simulink library "hysteresis_rods"  (R2016b)
settings: Solver=VariableStepAuto  StartTime=0.0  StopTime=10.0  RelTol=1e-3
undefined symbols (not defined in the file or in its folder): sim_params
libraries: hysteresis_curve x2, aerolibutil x1
settings Model: Creator=Sean  LastModifiedBy=bijan

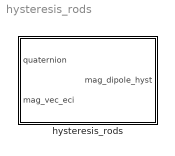
== system hysteresis_rods ==
  hysteresis_rods : Subsystem

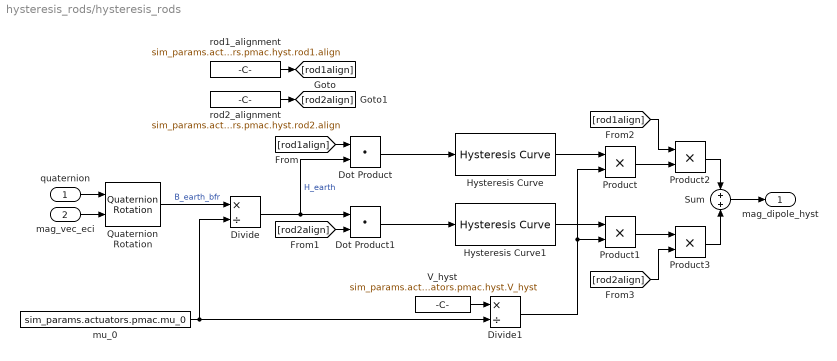
== system hysteresis_rods/hysteresis_rods ==
  quaternion : Inport
  mag_vec_eci : Inport  Port=2
  Divide : Product  Inputs=*/
  Divide1 : Product  Inputs=*/
  Dot Product : DotProduct  InputSameDT=on  OutDataTypeStr=Inherit: Inherit via internal rule
  Dot Product1 : DotProduct  InputSameDT=on  OutDataTypeStr=Inherit: Inherit via internal rule
  Hysteresis Curve : hysteresis_curve/Hysteresis Curve
  Hysteresis Curve1 : hysteresis_curve/Hysteresis Curve
  Product{,1..3} (4 alike) : Product
  Quaternion Rotation : aerolibutil/Quaternion Rotation
  Sum : Sum
  V_hyst : Constant  Value=sim_params.actuators.pmac.hyst.V_hyst
  mu_0 : Constant  Value=sim_params.actuators.pmac.mu_0
  rod1_alignment : Constant  Value=sim_params.actuators.pmac.hyst.rod1.align
  rod2_alignment : Constant  Value=sim_params.actuators.pmac.hyst.rod2.align
  mag_dipole_hyst : Outport
  wires:
  quaternion/1 -> Quaternion Rotation/1
  mag_vec_eci/1 -> Quaternion Rotation/2
  mu_0/1 -> Divide1/2, Divide/2
  Quaternion Rotation/1 -> Divide/1  "B_earth_bfr"
  V_hyst/1 -> Divide1/1
  Hysteresis Curve/1 -> Product/1
  Divide1/1 -> Product1/2, Product/2
  Divide/1 -> Dot Product1/1, Dot Product/2  "H_earth"
  Dot Product/1 -> Hysteresis Curve/1
  Dot Product1/1 -> Hysteresis Curve1/1
  Hysteresis Curve1/1 -> Product1/1
  rod1_alignment/1 -> [rod1align]
  [rod1align] -> Dot Product/1
  rod2_alignment/1 -> [rod2align]
  [rod2align] -> Dot Product1/2
  Product/1 -> Product2/2
  [rod1align] -> Product2/1
  Product1/1 -> Product3/1
  [rod2align] -> Product3/2
  Product2/1 -> Sum/1
  Product3/1 -> Sum/2
  Sum/1 -> mag_dipole_hyst/1
